simulink model "SensorSignals"  (R2024b)
settings: configuration reference "STM32H7_Config" (kept outside this file)
settings Model: DataDictionary=Master_Dictionary.sldd  EnableAccessToBaseWorkspace=off  Creator=torni  LastModifiedBy=oxbro
settings ConfigSetRef: SourceName=STM32H7_Config

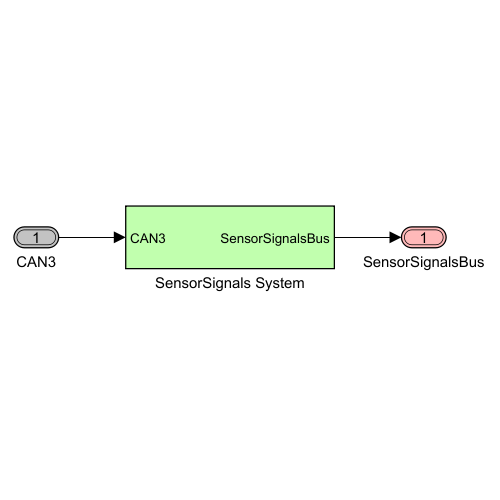
[thumbnail: Simulink's stored preview of the top-level diagram]
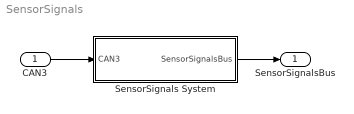
== system SensorSignals ==
  CAN3 : Inport  OutDataTypeStr=Bus: CAN3Bus
  SensorSignals System : Subsystem
  SensorSignalsBus : Outport  OutDataTypeStr=Bus: SensorSignalsBus  VectorParamsAs1DForOutWhenUnconnected=off
  wires:
  CAN3/1 -> SensorSignals System/1(CAN3)
  SensorSignals System/1(SensorSignalsBus) -> SensorSignalsBus/1

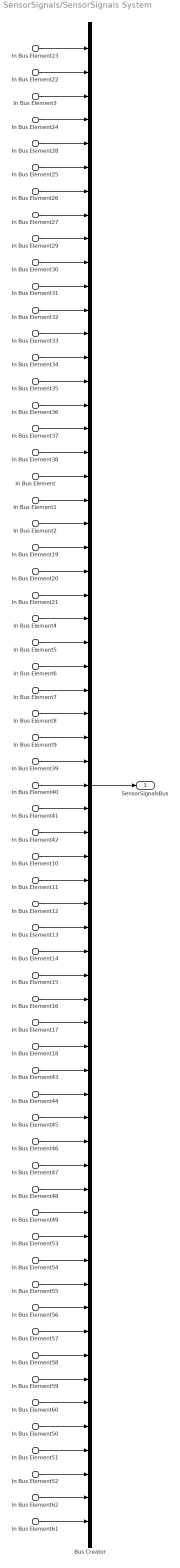
== system SensorSignals/SensorSignals System ==
  In Bus Element22 : Inport  PortName=CAN3  Element=DDU7_Analoge_1.pBrakeR
  In Bus Element23 : Inport  PortName=CAN3  Element=DDU7_Analoge_1.pBrakeF
  In Bus Element3 : Inport  PortName=CAN3  Element=DDU7_Analoge_1.VDamperPotentiometerFL
  In Bus Element24 : Inport  PortName=CAN3  Element=DDU7_Analoge_1.VDamperPotentiometerFR
  In Bus Element61 : Inport  PortName=CAN3  Element=DDU7_Analoge_1.VDamperPotentiometerRR
  In Bus Element62 : Inport  PortName=CAN3  Element=DDU7_Analoge_1.VDamperPotentiometerRL
  In Bus Element25 : Inport  PortName=CAN3  Element=DDU7_Analoge_2.VSteeringAngle
  In Bus Element28 : Inport  PortName=CAN3  Element=DDU7_Analoge_2.NDisplayNumberDDU7
  In Bus Element26 : Inport  PortName=CAN3  Element=DDU7_Analoge_2.VThrottlePedal1
  In Bus Element27 : Inport  PortName=CAN3  Element=DDU7_Analoge_2.VThrottlePedal2
  In Bus Element29 : Inport  PortName=CAN3  Element=SteeringWheelBus.BSteeringWheelButton1
  In Bus Element30 : Inport  PortName=CAN3  Element=SteeringWheelBus.BSteeringWheelButton2
  In Bus Element31 : Inport  PortName=CAN3  Element=SteeringWheelBus.BSteeringWheelButton3
  In Bus Element32 : Inport  PortName=CAN3  Element=SteeringWheelBus.BSteeringWheelButton4
  In Bus Element33 : Inport  PortName=CAN3  Element=SteeringWheelBus.BSteeringWheelButton5
  In Bus Element34 : Inport  PortName=CAN3  Element=SteeringWheelBus.BSteeringWheelButton6
  In Bus Element35 : Inport  PortName=CAN3  Element=SteeringWheelBus.BSteeringWheelButton7
  In Bus Element36 : Inport  PortName=CAN3  Element=SteeringWheelBus.BSteeringWheelButton8
  In Bus Element37 : Inport  PortName=CAN3  Element=SteeringWheelBus.VRegenPaddle1
  In Bus Element38 : Inport  PortName=CAN3  Element=SteeringWheelBus.VRegenPaddle2
  In Bus Element : Inport  PortName=CAN3  Element=PDM_Status_1.C1P01_Status
  In Bus Element1 : Inport  PortName=CAN3  Element=PDM_Status_1.C1P02_Status
  In Bus Element2 : Inport  PortName=CAN3  Element=PDM_Status_1.C1P03_Status
  In Bus Element19 : Inport  PortName=CAN3  Element=PDM_Status_1.C1P04_Status
  In Bus Element20 : Inport  PortName=CAN3  Element=PDM_Status_1.C1P07_Status
  In Bus Element21 : Inport  PortName=CAN3  Element=PDM_Status_1.C1P11_Status
  In Bus Element4 : Inport  PortName=CAN3  Element=PDM_Status_1.C1P12_Status
  In Bus Element5 : Inport  PortName=CAN3  Element=PDM_Status_1.C1P13_Status
  In Bus Element6 : Inport  PortName=CAN3  Element=PDM_Status_1.C1P25_Status
  In Bus Element7 : Inport  PortName=CAN3  Element=PDM_Status_1.C1P26_Status
  In Bus Element8 : Inport  PortName=CAN3  Element=PDM_Status_1.C1P28_Status
  In Bus Element9 : Inport  PortName=CAN3  Element=PDM_Status_1.C1P30_Status
  In Bus Element39 : Inport  PortName=CAN3  Element=PDM_Status_1.C1P31_Status
  In Bus Element40 : Inport  PortName=CAN3  Element=PDM_Status_1.C1P33_Status
  In Bus Element41 : Inport  PortName=CAN3  Element=PDM_Status_1.C1P34_Status
  In Bus Element42 : Inport  PortName=CAN3  Element=PDM_Status_1.C1P36_Status
  In Bus Element10 : Inport  PortName=CAN3  Element=PDM_Status_2.C1P37_Status
  In Bus Element11 : Inport  PortName=CAN3  Element=PDM_Status_2.C1P38_Status
  In Bus Element12 : Inport  PortName=CAN3  Element=PDM_Status_2.C2P01_Status
  In Bus Element13 : Inport  PortName=CAN3  Element=PDM_Status_2.C2P02_Status
  In Bus Element14 : Inport  PortName=CAN3  Element=PDM_Status_2.C2P03_Status
  In Bus Element15 : Inport  PortName=CAN3  Element=PDM_Status_2.C2P04_Status
  In Bus Element16 : Inport  PortName=CAN3  Element=PDM_Status_2.C2P05_Status
  In Bus Element17 : Inport  PortName=CAN3  Element=PDM_Status_2.C2P13_Status
  In Bus Element18 : Inport  PortName=CAN3  Element=PDM_Status_2.C2P25_Status
  In Bus Element43 : Inport  PortName=CAN3  Element=PDM_Status_2.C2P26_Status
  In Bus Element44 : Inport  PortName=CAN3  Element=PDM_Status_2.C2P27_Status
  In Bus Element45 : Inport  PortName=CAN3  Element=PDM_Status_2.C2P28_Status
  In Bus Element46 : Inport  PortName=CAN3  Element=PDM_Status_2.C2P29_Status
  In Bus Element47 : Inport  PortName=CAN3  Element=PDM_Status_2.C2P30_Status
  In Bus Element48 : Inport  PortName=CAN3  Element=PDM_Status_2.C2P31_Status
  In Bus Element49 : Inport  PortName=CAN3  Element=PDM_Status_2.C2P33_Status
  In Bus Element50 : Inport  PortName=CAN3  Element=PDM_Status_3.ILVSystem
  In Bus Element51 : Inport  PortName=CAN3  Element=PDM_Status_3.TLVSystem
  In Bus Element52 : Inport  PortName=CAN3  Element=PDM_Status_3.VLVSystem
  In Bus Element53 : Inport  PortName=CAN3  Element=PDM_Status_3.C1P16_Digital
  In Bus Element54 : Inport  PortName=CAN3  Element=PDM_Status_3.C1P17_Digital
  In Bus Element55 : Inport  PortName=CAN3  Element=PDM_Status_3.C2P17_Digital
  In Bus Element56 : Inport  PortName=CAN3  Element=PDM_Status_3.C2P18_Digital
  In Bus Element57 : Inport  PortName=CAN3  Element=PDM_Status_3.C2P35_Status
  In Bus Element58 : Inport  PortName=CAN3  Element=PDM_Status_3.C2P36_Status
  In Bus Element59 : Inport  PortName=CAN3  Element=PDM_Status_3.C2P37_Status
  In Bus Element60 : Inport  PortName=CAN3  Element=PDM_Status_3.C2P38_Status
  Bus Creator : BusCreator  Inputs=63  OutDataTypeStr=Bus: SensorSignalsBus
  SensorSignalsBus : Outport  OutDataTypeStr=Bus: SensorSignalsBus  VectorParamsAs1DForOutWhenUnconnected=off
  wires:
  Bus Creator/1 -> SensorSignalsBus/1
  In Bus Element52/1 -> Bus Creator/61
  In Bus Element51/1 -> Bus Creator/60
  In Bus Element50/1 -> Bus Creator/59
  In Bus Element60/1 -> Bus Creator/58
  In Bus Element59/1 -> Bus Creator/57
  In Bus Element58/1 -> Bus Creator/56
  In Bus Element57/1 -> Bus Creator/55
  In Bus Element56/1 -> Bus Creator/54
  In Bus Element55/1 -> Bus Creator/53
  In Bus Element54/1 -> Bus Creator/52
  In Bus Element53/1 -> Bus Creator/51
  In Bus Element49/1 -> Bus Creator/50
  In Bus Element48/1 -> Bus Creator/49
  In Bus Element47/1 -> Bus Creator/48
  In Bus Element23/1 -> Bus Creator/1
  In Bus Element22/1 -> Bus Creator/2
  In Bus Element24/1 -> Bus Creator/4
  In Bus Element3/1 -> Bus Creator/3
  In Bus Element27/1 -> Bus Creator/8
  In Bus Element26/1 -> Bus Creator/7
  In Bus Element28/1 -> Bus Creator/5
  In Bus Element25/1 -> Bus Creator/6
  In Bus Element29/1 -> Bus Creator/9
  In Bus Element30/1 -> Bus Creator/10
  In Bus Element31/1 -> Bus Creator/11
  In Bus Element32/1 -> Bus Creator/12
  In Bus Element33/1 -> Bus Creator/13
  In Bus Element34/1 -> Bus Creator/14
  In Bus Element35/1 -> Bus Creator/15
  In Bus Element36/1 -> Bus Creator/16
  In Bus Element37/1 -> Bus Creator/17
  In Bus Element38/1 -> Bus Creator/18
  In Bus Element/1 -> Bus Creator/19
  In Bus Element1/1 -> Bus Creator/20
  In Bus Element2/1 -> Bus Creator/21
  In Bus Element19/1 -> Bus Creator/22
  In Bus Element20/1 -> Bus Creator/23
  In Bus Element21/1 -> Bus Creator/24
  In Bus Element4/1 -> Bus Creator/25
  In Bus Element5/1 -> Bus Creator/26
  In Bus Element6/1 -> Bus Creator/27
  In Bus Element7/1 -> Bus Creator/28
  In Bus Element8/1 -> Bus Creator/29
  In Bus Element9/1 -> Bus Creator/30
  In Bus Element39/1 -> Bus Creator/31
  In Bus Element40/1 -> Bus Creator/32
  In Bus Element41/1 -> Bus Creator/33
  In Bus Element42/1 -> Bus Creator/34
  In Bus Element10/1 -> Bus Creator/35
  In Bus Element11/1 -> Bus Creator/36
  In Bus Element12/1 -> Bus Creator/37
  In Bus Element13/1 -> Bus Creator/38
  In Bus Element14/1 -> Bus Creator/39
  In Bus Element15/1 -> Bus Creator/40
  In Bus Element16/1 -> Bus Creator/41
  In Bus Element17/1 -> Bus Creator/42
  In Bus Element18/1 -> Bus Creator/43
  In Bus Element43/1 -> Bus Creator/44
  In Bus Element44/1 -> Bus Creator/45
  In Bus Element45/1 -> Bus Creator/46
  In Bus Element46/1 -> Bus Creator/47
  In Bus Element61/1 -> Bus Creator/63
  In Bus Element62/1 -> Bus Creator/62
